simulink library "aeroblk_lib_HL20"  (R2023a)
settings: Solver=ode45  StartTime=0.0  StopTime=10.0  RelTol=1e-3
values from neighbouring files (symbols this model uses):
  alpha_vec_Cn0 = [-10 -5 0 5 10 15 20 25 30]    [aeroblk_init_HL20.m]
  b_ref = 13.89/m2ft    (= 4.23367186452)    [aeroblk_init_HL20.m]
  beta_vec_Cn0 = [0 2 5 10]    [aeroblk_init_HL20.m]
  Clbeta = -0.00787    [aeroblk_init_HL20.m]
  Clda = temp(:,6)    [aeroblk_init_HL20.m]
  Clddf = temp(:,4)    [aeroblk_init_HL20.m]
  Cldr = temp(:,6)    [aeroblk_init_HL20.m]
  Clp = [-4.98 -6.0 -3.98 -5.79 -4.25 -4.99 -6.49 -6.19 -8.10 -8.72 -24.10]*1e-1    [aeroblk_init_HL20.m]
  Clr = [4.96 5.98 8.40 8.06 6.86 5.72 6.03 8.99 9.57 13.57 44.90]*1e-1    [aeroblk_init_HL20.m]
  Cm0 = reshape(temp(:,2),length(beta_vec_0),length(alpha_vec_0))    [aeroblk_init_HL20.m]
  Cmda = temp(:,2)    [aeroblk_init_HL20.m]
  Cmde = temp(:,2)    [aeroblk_init_HL20.m]
  Cmdfn = temp(:,2)    [aeroblk_init_HL20.m]
  Cmdfp = temp(:,2)    [aeroblk_init_HL20.m]
  Cmdr = temp(:,2)    [aeroblk_init_HL20.m]
  Cmq = [-2.03 -1.58 -1.16 -1.76 -1.76 -1.75 -1.74 -2.52 -2.99 -5.71 -8]*1e-1    [aeroblk_init_HL20.m]
  Cn0 = [0 0.46 1.15 2.30 ... (first row only)    [aeroblk_init_HL20.m]
  Cnda = temp(:,5)    [aeroblk_init_HL20.m]
  Cnddf = temp(:,3)    [aeroblk_init_HL20.m]
  Cndr = temp(:,5)    [aeroblk_init_HL20.m]
  Cnp = [3.81 3.53 2.19 2.44 1.79 1.67 2.01 2.22 3.07 3.79 8.50]*1e-1    [aeroblk_init_HL20.m]
  Cnr = [-7.94 -8.37 -9.21 -9.22 -8.67 -9.22 -9.46 -10.07 -10.90 -12.86 -20.41]*1e-1    [aeroblk_init_HL20.m]
  CX0 = -reshape(temp(:,3),length(beta_vec_0),length(alpha_vec_0))    [aeroblk_init_HL20.m]
  CXda = -temp(:,3)    [aeroblk_init_HL20.m]
  CXddf = temp(:,1)    [aeroblk_init_HL20.m]
  CXde = -temp(:,3)    [aeroblk_init_HL20.m]
  CXdfn = -temp(:,3)    [aeroblk_init_HL20.m]
  CXdfp = -temp(:,3)    [aeroblk_init_HL20.m]
  CXdr = -temp(:,3)    [aeroblk_init_HL20.m]
  CYbeta = -0.01242    [aeroblk_init_HL20.m]
  CYda = temp(:,4)    [aeroblk_init_HL20.m]
  CYddf = temp(:,2)    [aeroblk_init_HL20.m]
  CYdr = temp(:,4)    [aeroblk_init_HL20.m]
  CZ0 = -reshape(temp(:,1),length(beta_vec_0),length(alpha_vec_0))    [aeroblk_init_HL20.m]
  CZda = -temp(:,1)    [aeroblk_init_HL20.m]
  CZde = -temp(:,1)    [aeroblk_init_HL20.m]
  CZdfn = -temp(:,1)    [aeroblk_init_HL20.m]
  CZdfp = -temp(:,1)    [aeroblk_init_HL20.m]
  CZdr = -temp(:,1)    [aeroblk_init_HL20.m]
  d_ref = 28.24/m2ft    (= 8.60755172456)    [aeroblk_init_HL20.m]
  mass = massBody+massFuel    (= 11738.9844962)    [aeroblk_init_HL20.m]
  x_cg = 0.575*len_veh    (= 4.78635044684)    [aeroblk_init_HL20.m]
  x_ref = 0.54*len_veh    (= 4.49500737616)    [aeroblk_init_HL20.m]
undefined symbols (not defined in the file or in its folder): a_matrix, A_matrix, b_matrix, B_matrix, c_matrix, C_matrix, d_matrix, F, F_matrix, H_matrix, Kalpha, Kalpha_1, Kbeta, Kbeta_1, Kp, Kp_1, Kphi, Kphi_1, Kq, Kq_1, Kr, Kr_1, Light, MIL
libraries: aerolibschedule x4, aerolibconvert2 x3, aerolibasang x3, aerolibwind2 x3, shared6dof x1, aerolibatmos2 x1, aerolibadyn x1
(part 1 of 2)
Description:
  | HL-20 lifting body and controller library
settings Model: Creator=The MathWorks, Inc.  LastModifiedBy=The MathWorks, Inc.
settings SolverCC: AlgebraicLoopSolver=TrustRegion
settings DataIOCC: LimitDataPoints=on  SaveFormat=Array  SignalLoggingSaveFormat=ModelDataLogs  ReturnWorkspaceOutputs=off
settings OptimizationCC: BlockReduction=off  BooleanDataType=off  ReuseModelBlockBuffer=off  ExpressionDepthLimit=2147483647  LifeSpan=inf
settings DebuggingCC: SaveWithParameterizedLinksMsg=none  UnderspecifiedInitializationDetection=Classic  MergeDetectMultiDrivingBlocksExec=none  SignalResolutionControl=TryResolveAllWithWarning  FcnCallInpInsideContextMsg=warning  UnconnectedInputMsg=warning  UnconnectedOutputMsg=warning  UnconnectedLineMsg=warning  AllowSymbolicDim=off  StateNameClashWarn=warning  SFUnexpectedBacktrackingDiag=warning  SFNoUnconditionalDefaultTransitionDiag=warning  SFExecutionAtInitializationDiag=none  ArithmeticOperatorsInVariantConditions=warning
settings HardwareCC: ProdBitPerPointer=32  ProdBitPerSizeT=32  ProdBitPerPtrDiffT=32  ProdLargestAtomicFloat=None  ProdIntDivRoundTo=Undefined  ProdEndianess=Unspecified  ProdWordSize=32  ProdHWDeviceType=32-bit Generic  TargetUnknown=on
settings ModelReferenceCC: EnableRefExpFcnMdlSchedulingChecks=on  PropagateSignalLabelsOutOfModel=off
settings SFSimCC: SimUseLocalCustomCode=off  CustomCodeUndefinedFunction=UseInterfaceOnly
settings RTWCC: RTWUseLocalCustomCode=off
settings CodeAppCC: StateflowObjectComments=on
settings GRTTargetCC: TargetLangStandard=C89/C90 (ANSI)
settings ConfigComp: CovMetricSettings=dw  CovSaveCumulativeToWorkspaceVar=on  CovSaveSingleToWorkspaceVar=on  CovExternalEMLEnable=off

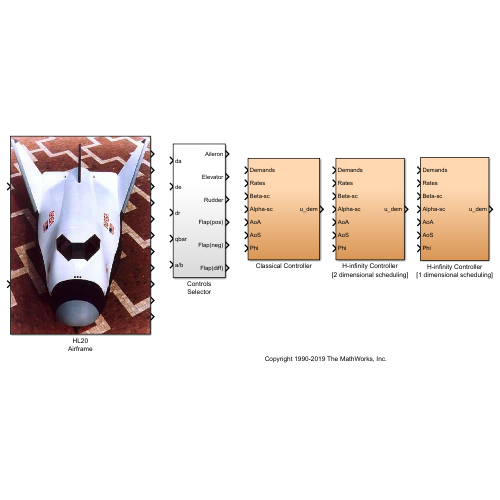
[thumbnail: Simulink's stored preview of the top-level diagram]
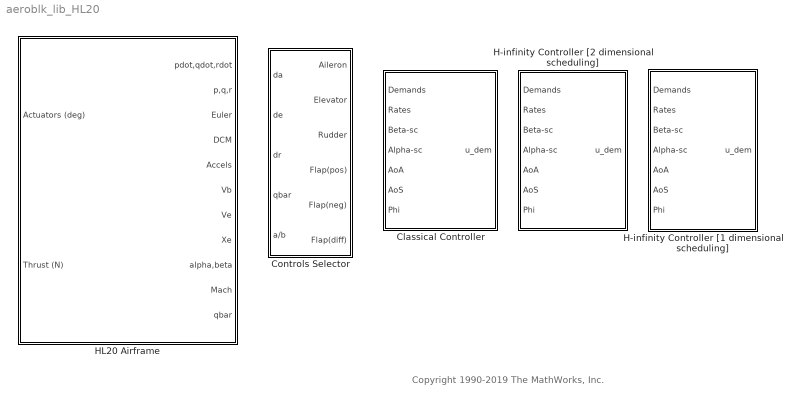
== system aeroblk_lib_HL20 ==
  note: Copyright 1990-2019 The MathWorks, Inc.
  Classical Controller : Subsystem
  Controls Selector : Subsystem
  H-infinity Controller [1 dimensional scheduling] : Subsystem
  H-infinity Controller [2 dimensional scheduling] : Subsystem
  HL20 Airframe : Subsystem
      mask Display: image('aeroblk_HL20pic.jpg')

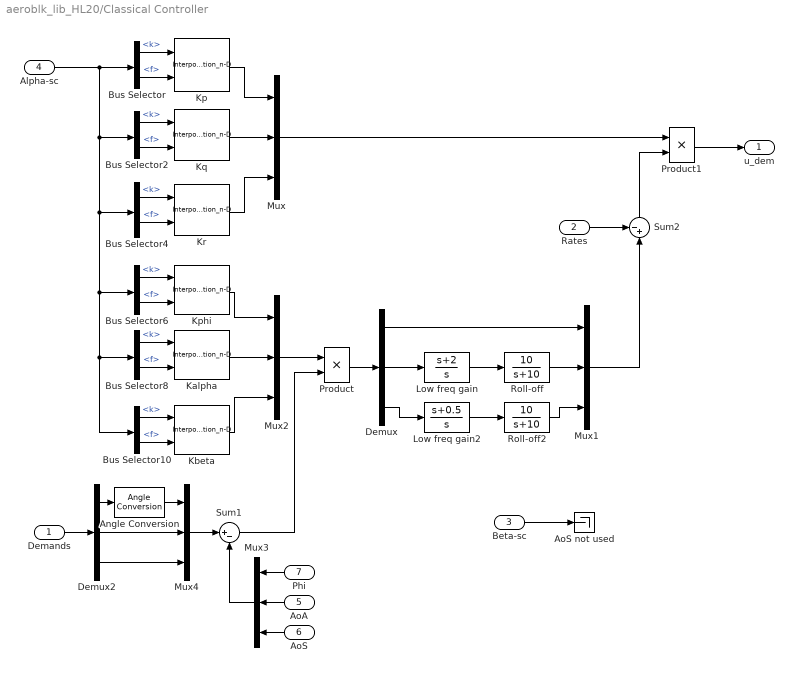
== system aeroblk_lib_HL20/Classical Controller ==
  Demands : Inport  Unit=deg  PortDimensions=3
  Rates : Inport  Port=2  Unit=rad/second  PortDimensions=3
  Beta-sc : Inport  Port=3
  Alpha-sc : Inport  Port=4
  AoA : Inport  Port=5  Unit=deg  PortDimensions=1
  AoS : Inport  Port=6  Unit=deg  PortDimensions=1
  Phi : Inport  Port=7  Unit=rad  PortDimensions=1
  Angle Conversion : aerolibconvert2/Angle Conversion  IU=deg  OU=rad
  AoS not used : Terminator
  Bus Selector{,2,4,6,8,10} (6 alike) : BusSelector  OutputSignals=k,f
  Demux : Demux  Outputs=3
      settings: DisplayOption=none
  Demux2 : Demux  Outputs=3
      settings: DisplayOption=none
  Kalpha : Interpolation_n-D  NumberOfTableDimensions=1  Table=Kalpha_1  RemoveProtectionIndex=on
      settings: InputPortMap=u0,u1
  Kbeta : Interpolation_n-D  NumberOfTableDimensions=1  Table=Kbeta_1  RemoveProtectionIndex=on
      settings: InputPortMap=u0,u1
  Kp : Interpolation_n-D  NumberOfTableDimensions=1  Table=Kp_1  RemoveProtectionIndex=on
      settings: InputPortMap=u0,u1
  Kphi : Interpolation_n-D  NumberOfTableDimensions=1  Table=Kphi_1  RemoveProtectionIndex=on
      settings: InputPortMap=u0,u1
  Kq : Interpolation_n-D  NumberOfTableDimensions=1  Table=Kq_1  RemoveProtectionIndex=on
      settings: InputPortMap=u0,u1
  Kr : Interpolation_n-D  NumberOfTableDimensions=1  Table=Kr_1  RemoveProtectionIndex=on
      settings: InputPortMap=u0,u1
  Low freq gain : TransferFcn  Numerator=[1 2]  Denominator=[1 0]
  Low freq gain2 : TransferFcn  Numerator=[1 0.5]  Denominator=[1 0]
  Mux{,1,3..4} (4 alike) : Mux  Inputs=[1,1,1]
  Mux2 : Mux  Inputs=3
  Product : Product  InputSameDT=on  SaturateOnIntegerOverflow=on  OutDataTypeStr=Inherit: Same as first input
  Product1 : Product  InputSameDT=on  SaturateOnIntegerOverflow=on  OutDataTypeStr=Inherit: Same as first input
  Roll-off : TransferFcn  Numerator=10  Denominator=[1 10]
  Roll-off2 : TransferFcn  Numerator=10  Denominator=[1 10]
  Sum1 : Sum  Inputs=|+-  InputSameDT=on  SaturateOnIntegerOverflow=on  OutDataTypeStr=Inherit: Same as first input
  Sum2 : Sum  Inputs=-+|  InputSameDT=on  SaturateOnIntegerOverflow=on  OutDataTypeStr=Inherit: Same as first input
  u_dem : Outport  OutputWhenDisabled=reset  InitialOutput=[0 0 0]  VectorParamsAs1DForOutWhenUnconnected=off
  wires:
  Beta-sc/1 -> AoS not used/1
  Product1/1 -> u_dem/1
  Mux4/1 -> Sum1/1
  Demux2/3 -> Mux4/3
  Demux2/2 -> Mux4/2
  Angle Conversion/1 -> Mux4/1
  Demux2/1 -> Angle Conversion/1
  Demands/1 -> Demux2/1
  Kphi/1 -> Mux2/1
  Kbeta/1 -> Mux2/3
  Kalpha/1 -> Mux2/2
  Mux1/1 -> Sum2/2
  Sum2/1 -> Product1/2
  Mux/1 -> Product1/1
  Rates/1 -> Sum2/1
  Demux/1 -> Mux1/1
  Roll-off2/1 -> Mux1/3
  Roll-off/1 -> Mux1/2
  Demux/3 -> Low freq gain2/1
  Demux/2 -> Low freq gain/1
  Product/1 -> Demux/1
  Sum1/1 -> Product/2
  Mux2/1 -> Product/1
  AoS/1 -> Mux3/3
  AoA/1 -> Mux3/2
  Phi/1 -> Mux3/1
  Mux3/1 -> Sum1/2
  Low freq gain/1 -> Roll-off/1
  Low freq gain2/1 -> Roll-off2/1
  Kr/1 -> Mux/3
  Kp/1 -> Mux/1
  Kq/1 -> Mux/2
  Bus Selector/1 -> Kp/1  "<k>"
  Bus Selector/2 -> Kp/2  "<f>"
  Bus Selector2/1 -> Kq/1  "<k>"
  Bus Selector2/2 -> Kq/2  "<f>"
  Bus Selector4/1 -> Kr/1  "<k>"
  Bus Selector4/2 -> Kr/2  "<f>"
  Bus Selector6/1 -> Kphi/1  "<k>"
  Bus Selector6/2 -> Kphi/2  "<f>"
  Bus Selector8/1 -> Kalpha/1  "<k>"
  Bus Selector10/1 -> Kbeta/1  "<k>"
  Bus Selector10/2 -> Kbeta/2  "<f>"
  Bus Selector8/2 -> Kalpha/2  "<f>"
  Alpha-sc/1 -> Bus Selector/1, Bus Selector2/1, Bus Selector4/1, Bus Selector6/1, Bus Selector8/1, Bus Selector10/1

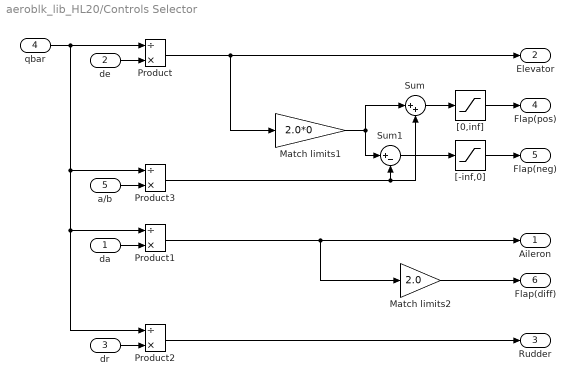
== system aeroblk_lib_HL20/Controls Selector ==
  da : Inport
  de : Inport  Port=2
  dr : Inport  Port=3
  qbar : Inport  Port=4  Unit=pascal
  a/b : Inport  Port=5
  Match limits1 : Gain  Gain=2.0*0  SaturateOnIntegerOverflow=on  OutDataTypeStr=Inherit: Same as input  ParamDataTypeStr=Inherit: Same as input
  Match limits2 : Gain  Gain=2.0  SaturateOnIntegerOverflow=on  OutDataTypeStr=Inherit: Same as input  ParamDataTypeStr=Inherit: Same as input
  Product{,1..3} (4 alike) : Product  Inputs=/*  InputSameDT=on  SaturateOnIntegerOverflow=on  OutDataTypeStr=Inherit: Same as first input
  Sum : Sum  Inputs=|++  InputSameDT=on  SaturateOnIntegerOverflow=on  OutDataTypeStr=Inherit: Same as first input
  Sum1 : Sum  Inputs=|+-  InputSameDT=on  SaturateOnIntegerOverflow=on  OutDataTypeStr=Inherit: Same as first input
  "[-inf,0]" : Saturate  UpperLimit=0  LowerLimit=-inf
  "[0,inf]" : Saturate  UpperLimit=inf  LowerLimit=0
  Aileron : Outport  Unit=deg  VectorParamsAs1DForOutWhenUnconnected=off
  Elevator : Outport  Port=2  Unit=deg  VectorParamsAs1DForOutWhenUnconnected=off
  Rudder : Outport  Port=3  Unit=deg  VectorParamsAs1DForOutWhenUnconnected=off
  Flap(pos) : Outport  Port=4  Unit=deg  VectorParamsAs1DForOutWhenUnconnected=off
  Flap(neg) : Outport  Port=5  Unit=deg  VectorParamsAs1DForOutWhenUnconnected=off
  Flap(diff) : Outport  Port=6  Unit=deg  VectorParamsAs1DForOutWhenUnconnected=off
  wires:
  qbar/1 -> Product/1, Product2/1, Product1/1, Product3/1
  de/1 -> Product/2
  Product2/1 -> Rudder/1
  dr/1 -> Product2/2
  da/1 -> Product1/2
  Product1/1 -> Match limits2/1, Aileron/1
  Product/1 -> Elevator/1, Match limits1/1
  Match limits1/1 -> Sum/1, Sum1/1
  "[-inf,0]"/1 -> Flap(neg)/1
  "[0,inf]"/1 -> Flap(pos)/1
  Match limits2/1 -> Flap(diff)/1
  a/b/1 -> Product3/2
  Sum/1 -> "[0,inf]"/1
  Sum1/1 -> "[-inf,0]"/1
  Product3/1 -> Sum1/2, Sum/2

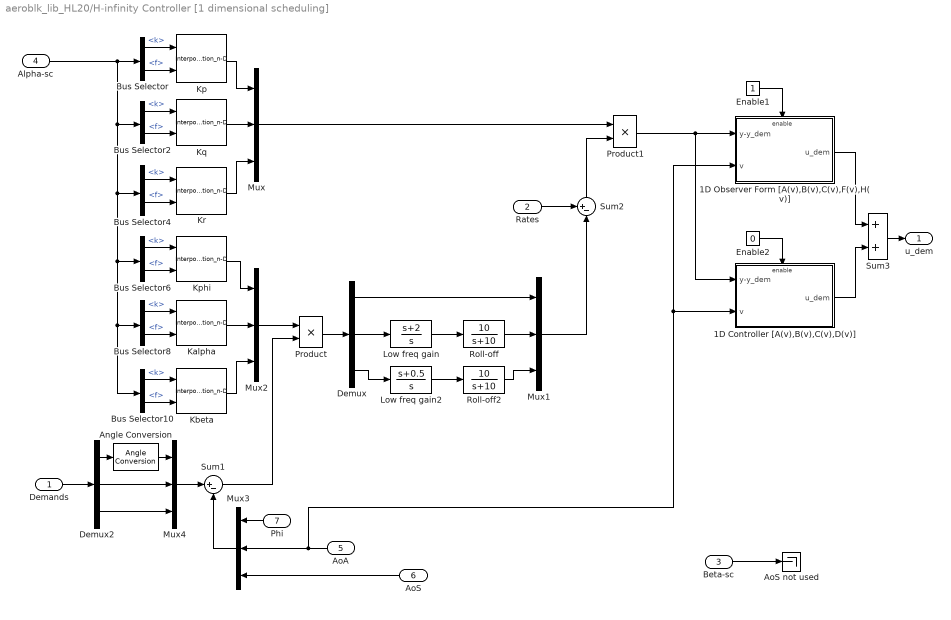
== system aeroblk_lib_HL20/H-infinity Controller [1 dimensional scheduling] ==
  Demands : Inport  Unit=deg  PortDimensions=3
  Rates : Inport  Port=2  Unit=rad/second  PortDimensions=3
  Beta-sc : Inport  Port=3
  Alpha-sc : Inport  Port=4
  AoA : Inport  Port=5  Unit=deg  PortDimensions=1
  AoS : Inport  Port=6  Unit=deg  PortDimensions=1
  Phi : Inport  Port=7  Unit=radian  PortDimensions=1
  1D Controller [A(v),B(v),C(v),D(v)] : Subsystem  TreatAsAtomicUnit=on
  1D Observer Form [A(v),B(v),C(v),F(v),H(v)] : Subsystem  TreatAsAtomicUnit=on
  Angle Conversion : aerolibconvert2/Angle Conversion  IU=deg  OU=rad
  AoS not used : Terminator
  Bus Selector{,2,4,6,8,10} (6 alike) : BusSelector  OutputSignals=k,f
  Demux : Demux  Outputs=3
      settings: DisplayOption=none
  Demux2 : Demux  Outputs=3
      settings: DisplayOption=none
  Enable1 : Constant
  Enable2 : Constant  Value=0
  Kalpha : Interpolation_n-D  NumberOfTableDimensions=1  Table=Kalpha_1  RemoveProtectionIndex=on
      settings: InputPortMap=u0,u1
  Kbeta : Interpolation_n-D  NumberOfTableDimensions=1  Table=Kbeta_1  RemoveProtectionIndex=on
      settings: InputPortMap=u0,u1
  Kp : Interpolation_n-D  NumberOfTableDimensions=1  Table=Kp_1  RemoveProtectionIndex=on
      settings: InputPortMap=u0,u1
  Kphi : Interpolation_n-D  NumberOfTableDimensions=1  Table=Kphi_1  RemoveProtectionIndex=on
      settings: InputPortMap=u0,u1
  Kq : Interpolation_n-D  NumberOfTableDimensions=1  Table=Kq_1  RemoveProtectionIndex=on
      settings: InputPortMap=u0,u1
  Kr : Interpolation_n-D  NumberOfTableDimensions=1  Table=Kr_1  RemoveProtectionIndex=on
      settings: InputPortMap=u0,u1
  Low freq gain : TransferFcn  Numerator=[1 2]  Denominator=[1 0]
  Low freq gain2 : TransferFcn  Numerator=[1 0.5]  Denominator=[1 0]
  Mux{,1,3..4} (4 alike) : Mux  Inputs=[1,1,1]
  Mux2 : Mux  Inputs=3
  Product : Product  InputSameDT=on  SaturateOnIntegerOverflow=on  OutDataTypeStr=Inherit: Same as first input
  Product1 : Product  InputSameDT=on  SaturateOnIntegerOverflow=on  OutDataTypeStr=Inherit: Same as first input
  Roll-off : TransferFcn  Numerator=10  Denominator=[1 10]
  Roll-off2 : TransferFcn  Numerator=10  Denominator=[1 10]
  Sum1 : Sum  Inputs=|+-  InputSameDT=on  SaturateOnIntegerOverflow=on  OutDataTypeStr=Inherit: Same as first input
  Sum2 : Sum  Inputs=+-|  InputSameDT=on  SaturateOnIntegerOverflow=on  OutDataTypeStr=Inherit: Same as first input
  Sum3 : Sum  InputSameDT=on  SaturateOnIntegerOverflow=on  OutDataTypeStr=Inherit: Same as first input
  u_dem : Outport  OutputWhenDisabled=reset  InitialOutput=[0 0 0]  VectorParamsAs1DForOutWhenUnconnected=off
  wires:
  Beta-sc/1 -> AoS not used/1
  Mux4/1 -> Sum1/1
  Demux2/3 -> Mux4/3
  Demux2/2 -> Mux4/2
  Angle Conversion/1 -> Mux4/1
  Demux2/1 -> Angle Conversion/1
  Demands/1 -> Demux2/1
  Mux1/1 -> Sum2/2
  Sum2/1 -> Product1/2
  Mux/1 -> Product1/1
  Rates/1 -> Sum2/1
  Demux/1 -> Mux1/1
  Roll-off2/1 -> Mux1/3
  Roll-off/1 -> Mux1/2
  Demux/3 -> Low freq gain2/1
  Demux/2 -> Low freq gain/1
  Product/1 -> Demux/1
  Sum1/1 -> Product/2
  Mux2/1 -> Product/1
  AoS/1 -> Mux3/3
  AoA/1 -> 1D Observer Form [A(v),B(v),C(v),F(v),H(v)]/2(v), 1D Controller [A(v),B(v),C(v),D(v)]/2(v), Mux3/2
  Phi/1 -> Mux3/1
  Mux3/1 -> Sum1/2
  Low freq gain/1 -> Roll-off/1
  Low freq gain2/1 -> Roll-off2/1
  Alpha-sc/1 -> Bus Selector8/1, Bus Selector10/1, Bus Selector6/1, Bus Selector4/1, Bus Selector2/1, Bus Selector/1
  Product1/1 -> 1D Observer Form [A(v),B(v),C(v),F(v),H(v)]/1(y-y_dem), 1D Controller [A(v),B(v),C(v),D(v)]/1(y-y_dem)
  Enable1/1 -> 1D Observer Form [A(v),B(v),C(v),F(v),H(v)]/Enable
  Enable2/1 -> 1D Controller [A(v),B(v),C(v),D(v)]/Enable
  1D Observer Form [A(v),B(v),C(v),F(v),H(v)]/1(u_dem) -> Sum3/1
  1D Controller [A(v),B(v),C(v),D(v)]/1(u_dem) -> Sum3/2
  Sum3/1 -> u_dem/1
  Bus Selector8/2 -> Kalpha/2  "<f>"
  Bus Selector10/2 -> Kbeta/2  "<f>"
  Bus Selector10/1 -> Kbeta/1  "<k>"
  Bus Selector8/1 -> Kalpha/1  "<k>"
  Bus Selector6/2 -> Kphi/2  "<f>"
  Bus Selector6/1 -> Kphi/1  "<k>"
  Bus Selector4/2 -> Kr/2  "<f>"
  Bus Selector4/1 -> Kr/1  "<k>"
  Bus Selector2/2 -> Kq/2  "<f>"
  Bus Selector2/1 -> Kq/1  "<k>"
  Bus Selector/2 -> Kp/2  "<f>"
  Bus Selector/1 -> Kp/1  "<k>"
  Kp/1 -> Mux/1
  Kq/1 -> Mux/2
  Kr/1 -> Mux/3
  Kphi/1 -> Mux2/1
  Kbeta/1 -> Mux2/3
  Kalpha/1 -> Mux2/2

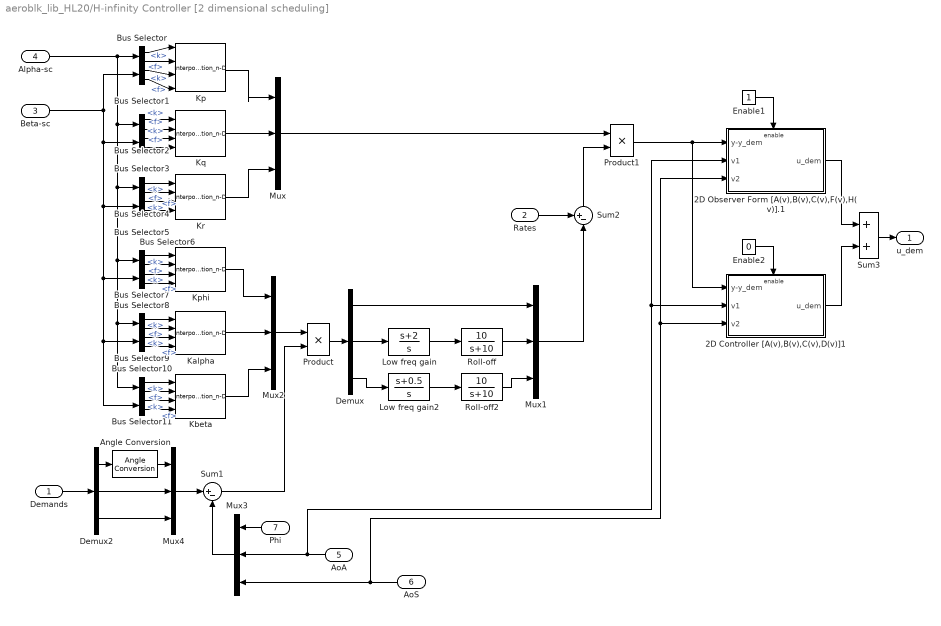
== system aeroblk_lib_HL20/H-infinity Controller [2 dimensional scheduling] ==
  Demands : Inport  Unit=degree  PortDimensions=3
  Rates : Inport  Port=2  Unit=rad/second  PortDimensions=3
  Beta-sc : Inport  Port=3
  Alpha-sc : Inport  Port=4
  AoA : Inport  Port=5  Unit=deg  PortDimensions=1
  AoS : Inport  Port=6  Unit=deg  PortDimensions=1
  Phi : Inport  Port=7  Unit=radian  PortDimensions=1
  2D Controller [A(v),B(v),C(v),D(v)]1 : Subsystem  TreatAsAtomicUnit=on
  2D Observer Form [A(v),B(v),C(v),F(v),H(v)].1 : Subsystem  TreatAsAtomicUnit=on
  Angle Conversion : aerolibconvert2/Angle Conversion  IU=deg  OU=rad
  Bus Selector{,1..11} (12 alike) : BusSelector  OutputSignals=k,f
  Demux : Demux  Outputs=3
      settings: DisplayOption=none
  Demux2 : Demux  Outputs=3
      settings: DisplayOption=none
  Enable1 : Constant
  Enable2 : Constant  Value=0
  Kalpha : Interpolation_n-D  Table=Kalpha  RemoveProtectionIndex=on
  Kbeta : Interpolation_n-D  Table=Kbeta  RemoveProtectionIndex=on
  Kp : Interpolation_n-D  Table=Kp  RemoveProtectionIndex=on
  Kphi : Interpolation_n-D  Table=Kphi  RemoveProtectionIndex=on
  Kq : Interpolation_n-D  Table=Kq  RemoveProtectionIndex=on
  Kr : Interpolation_n-D  Table=Kr  RemoveProtectionIndex=on
  Low freq gain : TransferFcn  Numerator=[1 2]  Denominator=[1 0]
  Low freq gain2 : TransferFcn  Numerator=[1 0.5]  Denominator=[1 0]
  Mux{,1,3..4} (4 alike) : Mux  Inputs=[1,1,1]
  Mux2 : Mux  Inputs=3
  Product : Product  InputSameDT=on  SaturateOnIntegerOverflow=on  OutDataTypeStr=Inherit: Same as first input
  Product1 : Product  InputSameDT=on  SaturateOnIntegerOverflow=on  OutDataTypeStr=Inherit: Same as first input
  Roll-off : TransferFcn  Numerator=10  Denominator=[1 10]
  Roll-off2 : TransferFcn  Numerator=10  Denominator=[1 10]
  Sum1 : Sum  Inputs=|+-  InputSameDT=on  SaturateOnIntegerOverflow=on  OutDataTypeStr=Inherit: Same as first input
  Sum2 : Sum  Inputs=+-|  InputSameDT=on  SaturateOnIntegerOverflow=on  OutDataTypeStr=Inherit: Same as first input
  Sum3 : Sum  InputSameDT=on  SaturateOnIntegerOverflow=on  OutDataTypeStr=Inherit: Same as first input
  u_dem : Outport  OutputWhenDisabled=reset  InitialOutput=[0 0 0]  VectorParamsAs1DForOutWhenUnconnected=off
  wires:
  Sum3/1 -> u_dem/1
  2D Controller [A(v),B(v),C(v),D(v)]1/1(u_dem) -> Sum3/2
  2D Observer Form [A(v),B(v),C(v),F(v),H(v)].1/1(u_dem) -> Sum3/1
  Enable2/1 -> 2D Controller [A(v),B(v),C(v),D(v)]1/Enable
  Enable1/1 -> 2D Observer Form [A(v),B(v),C(v),F(v),H(v)].1/Enable
  Product1/1 -> 2D Observer Form [A(v),B(v),C(v),F(v),H(v)].1/1(y-y_dem), 2D Controller [A(v),B(v),C(v),D(v)]1/1(y-y_dem)
  Beta-sc/1 -> Bus Selector9/1, Bus Selector11/1, Bus Selector7/1, Bus Selector5/1, Bus Selector3/1, Bus Selector1/1
  Alpha-sc/1 -> Bus Selector8/1, Bus Selector10/1, Bus Selector6/1, Bus Selector4/1, Bus Selector2/1, Bus Selector/1
  Kq/1 -> Mux/2
  Kp/1 -> Mux/1
  Kr/1 -> Mux/3
  Low freq gain2/1 -> Roll-off2/1
  Low freq gain/1 -> Roll-off/1
  Mux3/1 -> Sum1/2
  Phi/1 -> Mux3/1
  AoA/1 -> 2D Observer Form [A(v),B(v),C(v),F(v),H(v)].1/2(v1), 2D Controller [A(v),B(v),C(v),D(v)]1/2(v1), Mux3/2
  AoS/1 -> 2D Observer Form [A(v),B(v),C(v),F(v),H(v)].1/3(v2), 2D Controller [A(v),B(v),C(v),D(v)]1/3(v2), Mux3/3
  Mux2/1 -> Product/1
  Sum1/1 -> Product/2
  Product/1 -> Demux/1
  Demux/2 -> Low freq gain/1
  Demux/3 -> Low freq gain2/1
  Roll-off/1 -> Mux1/2
  Roll-off2/1 -> Mux1/3
  Demux/1 -> Mux1/1
  Rates/1 -> Sum2/1
  Mux/1 -> Product1/1
  Sum2/1 -> Product1/2
  Mux1/1 -> Sum2/2
  Kalpha/1 -> Mux2/2
  Kbeta/1 -> Mux2/3
  Kphi/1 -> Mux2/1
  Demands/1 -> Demux2/1
  Demux2/1 -> Angle Conversion/1
  Angle Conversion/1 -> Mux4/1
  Demux2/2 -> Mux4/2
  Demux2/3 -> Mux4/3
  Mux4/1 -> Sum1/1
  Bus Selector/1 -> Kp/1  "<k>"
  Bus Selector/2 -> Kp/2  "<f>"
  Bus Selector1/1 -> Kp/3  "<k>"
  Bus Selector1/2 -> Kp/4  "<f>"
  Bus Selector2/1 -> Kq/1  "<k>"
  Bus Selector2/2 -> Kq/2  "<f>"
  Bus Selector3/1 -> Kq/3  "<k>"
  Bus Selector3/2 -> Kq/4  "<f>"
  Bus Selector4/1 -> Kr/1  "<k>"
  Bus Selector4/2 -> Kr/2  "<f>"
  Bus Selector5/1 -> Kr/3  "<k>"
  Bus Selector5/2 -> Kr/4  "<f>"
  Bus Selector6/1 -> Kphi/1  "<k>"
  Bus Selector6/2 -> Kphi/2  "<f>"
  Bus Selector7/1 -> Kphi/3  "<k>"
  Bus Selector7/2 -> Kphi/4  "<f>"
  Bus Selector8/1 -> Kalpha/1  "<k>"
  Bus Selector8/2 -> Kalpha/2  "<f>"
  Bus Selector9/1 -> Kalpha/3  "<k>"
  Bus Selector9/2 -> Kalpha/4  "<f>"
  Bus Selector10/1 -> Kbeta/1  "<k>"
  Bus Selector10/2 -> Kbeta/2  "<f>"
  Bus Selector11/1 -> Kbeta/3  "<k>"
  Bus Selector11/2 -> Kbeta/4  "<f>"

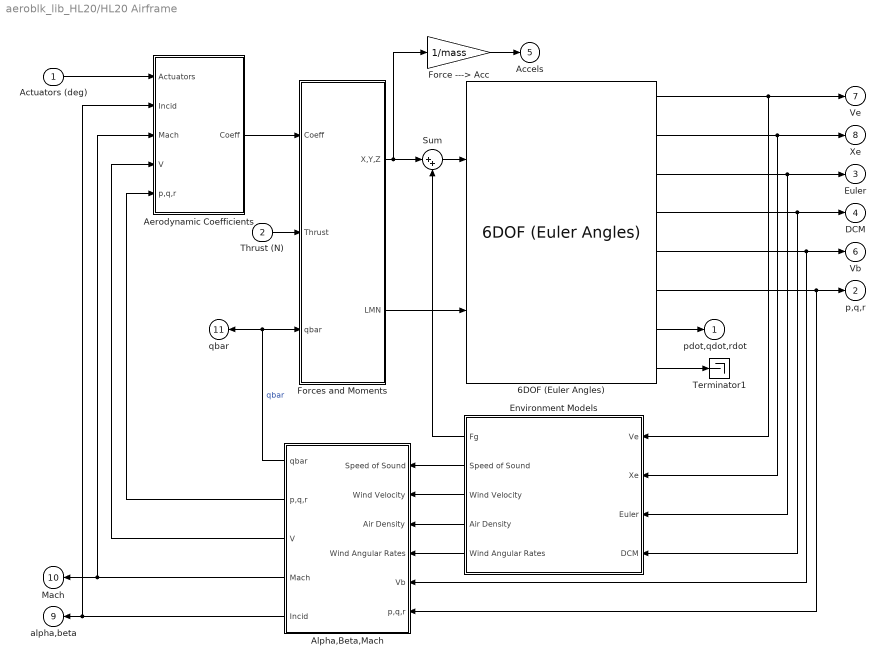
== system aeroblk_lib_HL20/HL20 Airframe ==
  Actuators (deg) : Inport  Unit=deg
  Thrust (N) : Inport  Port=2  Unit=N
  6DOF (Euler Angles) : shared6dof/6DOF (Euler Angles)  units=Metric (MKS)  mtype=Fixed  rep=Euler Angles  xme_0=xme_0  Vm_0=Vmw  eul_0=Euler_0  pm_0=pm_0  mass_0=mass  mass_e=0.5  mass_f=2.0  inertia=Inertia  inertia_e=eye(3)  inertia_f=2*eye(3)  k_quat=1.0  vre_flag=on  abi_flag=off  aMode=aMode  xme_statename=''  Vm_statename=''  eul_statename=''  quat_statename=''  pm_statename=''  mass_statename=''
  Aerodynamic Coefficients : Subsystem
  Alpha,Beta,Mach : Subsystem
  Environment Models : Subsystem
  Force ---> Acc : Gain  Gain=1/mass  SaturateOnIntegerOverflow=on  OutDataTypeStr=Inherit: Same as input  ParamDataTypeStr=Inherit: Same as input
  Forces and Moments : Subsystem
  Sum : Sum  Inputs=|++  InputSameDT=on  SaturateOnIntegerOverflow=on  OutDataTypeStr=Inherit: Same as first input
  Terminator1 : Terminator
  pdot,qdot,rdot : Outport  Unit=rad/s^2  InitialOutput=0  VectorParamsAs1DForOutWhenUnconnected=off
  p,q,r : Outport  Port=2  Unit=rad/second  InitialOutput=0  VectorParamsAs1DForOutWhenUnconnected=off
  Euler : Outport  Port=3  Unit=rad  InitialOutput=0  VectorParamsAs1DForOutWhenUnconnected=off
  DCM : Outport  Port=4  InitialOutput=0  VectorParamsAs1DForOutWhenUnconnected=off
  Accels : Outport  Port=5  Unit=m/s^2  InitialOutput=0  VectorParamsAs1DForOutWhenUnconnected=off
  Vb : Outport  Port=6  Unit=m/second  InitialOutput=0  VectorParamsAs1DForOutWhenUnconnected=off
  Ve : Outport  Port=7  Unit=m/s  InitialOutput=0  VectorParamsAs1DForOutWhenUnconnected=off
  Xe : Outport  Port=8  Unit=meter  InitialOutput=0  VectorParamsAs1DForOutWhenUnconnected=off
  alpha,beta : Outport  Port=9  Unit=rad  InitialOutput=0  VectorParamsAs1DForOutWhenUnconnected=off
  Mach : Outport  Port=10  InitialOutput=0  VectorParamsAs1DForOutWhenUnconnected=off
  qbar : Outport  Port=11  Unit=Pa  InitialOutput=0  VectorParamsAs1DForOutWhenUnconnected=off
  wires:
  Environment Models/5(Wind Angular Rates) -> Alpha,Beta,Mach/4(Wind Angular Rates)
  Alpha,Beta,Mach/2("p,q,r ") -> Aerodynamic Coefficients/5(p,q,r)
  Alpha,Beta,Mach/4(Mach) -> Mach/1, Aerodynamic Coefficients/3(Mach)
  Alpha,Beta,Mach/3(V) -> Aerodynamic Coefficients/4(V)
  Actuators (deg)/1 -> Aerodynamic Coefficients/1(Actuators)
  Force ---> Acc/1 -> Accels/1
  Environment Models/1(Fg) -> Sum/2
  Sum/1 -> 6DOF (Euler Angles)/1
  Forces and Moments/1(X,Y,Z) -> Sum/1, Force ---> Acc/1
  Alpha,Beta,Mach/1(qbar) -> qbar/1, Forces and Moments/3(qbar)  "qbar"
  Forces and Moments/2(LMN) -> 6DOF (Euler Angles)/2
  Environment Models/4(Air Density) -> Alpha,Beta,Mach/3(Air Density)
  Environment Models/2(Speed of Sound) -> Alpha,Beta,Mach/1(Speed of Sound)
  6DOF (Euler Angles)/5 -> Vb/1, Alpha,Beta,Mach/5(Vb)
  Environment Models/3(Wind Velocity) -> Alpha,Beta,Mach/2(Wind Velocity)
  Aerodynamic Coefficients/1(Coeff) -> Forces and Moments/1(Coeff)
  Alpha,Beta,Mach/5(Incid) -> Aerodynamic Coefficients/2(Incid), alpha,beta/1
  6DOF (Euler Angles)/3 -> Euler/1, Environment Models/3(Euler)
  6DOF (Euler Angles)/4 -> Environment Models/4(DCM), DCM/1
  6DOF (Euler Angles)/7 -> pdot,qdot,rdot/1
  Thrust (N)/1 -> Forces and Moments/2(Thrust)
  6DOF (Euler Angles)/6 -> Alpha,Beta,Mach/6(p,q,r), p,q,r/1
  6DOF (Euler Angles)/2 -> Xe/1, Environment Models/2(Xe)
  6DOF (Euler Angles)/1 -> Ve/1, Environment Models/1(Ve)
  6DOF (Euler Angles)/8 -> Terminator1/1

== system aeroblk_lib_HL20/H-infinity Controller [1 dimensional scheduling]/1D Controller [A(v),B(v),C(v),D(v)] ==
  y-y_dem : Inport  PortDimensions=3
  v : Inport  Port=2  PortDimensions=1
  Enable : EnablePort
  -1 : Gain  Gain=-1  SaturateOnIntegerOverflow=on  OutDataTypeStr=Inherit: Same as input  ParamDataTypeStr=Inherit: Same as input
  1D Controller [A(v),B(v),C(v),D(v)] : aerolibschedule/1D Controller [A(v),B(v),C(v),D(v)]  A=squeeze(a_matrix(:,:,:,3))  B=squeeze(b_matrix(:,:,:,3))  C=squeeze(c_matrix(:,:,:,3))  D=squeeze(d_matrix(:,:,:,3))  AoA_vec=a_vec  x_initial=0
  u_dem : Outport  OutputWhenDisabled=reset  InitialOutput=[0 0 0]  VectorParamsAs1DForOutWhenUnconnected=off
  wires:
  y-y_dem/1 -> -1/1
  -1/1 -> 1D Controller [A(v),B(v),C(v),D(v)]/1
  1D Controller [A(v),B(v),C(v),D(v)]/1 -> u_dem/1
  v/1 -> 1D Controller [A(v),B(v),C(v),D(v)]/2

== system aeroblk_lib_HL20/H-infinity Controller [1 dimensional scheduling]/1D Observer Form [A(v),B(v),C(v),F(v),H(v)] ==
  y-y_dem : Inport  PortDimensions=3
  v : Inport  Port=2  PortDimensions=1
  Enable : EnablePort
  1D Observer Form [A(v),B(v),C(v),F(v),H(v)] : aerolibschedule/1D Observer Form [A(v),B(v),C(v),F(v),H(v)]  A=squeeze(A_matrix(:,:,:,3))  B=squeeze(B_matrix(:,:,:,3))  C=squeeze(C_matrix(:,:,:,3))  F=squeeze(F_matrix(:,:,:,3))  H=squeeze(H_matrix(:,:,:,3))  AoA_vec=a_vec  x_initial=0
  Signal Specification : SignalSpecification  Dimensions=3
  u_dem : Outport  OutputWhenDisabled=reset  InitialOutput=[0 0 0]  VectorParamsAs1DForOutWhenUnconnected=off
  wires:
  y-y_dem/1 -> 1D Observer Form [A(v),B(v),C(v),F(v),H(v)]/1
  v/1 -> 1D Observer Form [A(v),B(v),C(v),F(v),H(v)]/2
  1D Observer Form [A(v),B(v),C(v),F(v),H(v)]/1 -> Signal Specification/1
  Signal Specification/1 -> 1D Observer Form [A(v),B(v),C(v),F(v),H(v)]/3, u_dem/1

== system aeroblk_lib_HL20/H-infinity Controller [2 dimensional scheduling]/2D Controller [A(v),B(v),C(v),D(v)]1 ==
  y-y_dem : Inport  PortDimensions=3
  v1 : Inport  Port=2  PortDimensions=1
  v2 : Inport  Port=3  PortDimensions=1
  Enable : EnablePort
  -1 : Gain  Gain=-1  SaturateOnIntegerOverflow=on  OutDataTypeStr=Inherit: Same as input  ParamDataTypeStr=Inherit: Same as input
  2D Controller [A(v),B(v),C(v),D(v)]1 : aerolibschedule/2D Controller [A(v),B(v),C(v),D(v)]  A=a_matrix  B=b_matrix  C=c_matrix  D=d_matrix  AoA_vec=a_vec  Mach_vec=b_vec  x_initial=0
  u_dem : Outport  OutputWhenDisabled=reset  InitialOutput=[0 0 0]  VectorParamsAs1DForOutWhenUnconnected=off
  wires:
  v2/1 -> 2D Controller [A(v),B(v),C(v),D(v)]1/3
  v1/1 -> 2D Controller [A(v),B(v),C(v),D(v)]1/2
  2D Controller [A(v),B(v),C(v),D(v)]1/1 -> u_dem/1
  -1/1 -> 2D Controller [A(v),B(v),C(v),D(v)]1/1
  y-y_dem/1 -> -1/1

== system aeroblk_lib_HL20/H-infinity Controller [2 dimensional scheduling]/2D Observer Form [A(v),B(v),C(v),F(v),H(v)].1 ==
  y-y_dem : Inport  PortDimensions=3
  v1 : Inport  Port=2  PortDimensions=1
  v2 : Inport  Port=3  PortDimensions=1
  Enable : EnablePort
  2D Observer Form [A(v),B(v),C(v),F(v),H(v)] : aerolibschedule/2D Observer Form [A(v),B(v),C(v),F(v),H(v)]  A=A_matrix  B=B_matrix  C=C_matrix  F=F_matrix  H=H_matrix  AoA_vec=a_vec  Mach_vec=b_vec  x_initial=0
  Signal Specification : SignalSpecification  Dimensions=3
  u_dem : Outport  OutputWhenDisabled=reset  InitialOutput=[0 0 0]  VectorParamsAs1DForOutWhenUnconnected=off
  wires:
  Signal Specification/1 -> 2D Observer Form [A(v),B(v),C(v),F(v),H(v)]/4, u_dem/1
  2D Observer Form [A(v),B(v),C(v),F(v),H(v)]/1 -> Signal Specification/1
  v2/1 -> 2D Observer Form [A(v),B(v),C(v),F(v),H(v)]/3
  v1/1 -> 2D Observer Form [A(v),B(v),C(v),F(v),H(v)]/2
  y-y_dem/1 -> 2D Observer Form [A(v),B(v),C(v),F(v),H(v)]/1

== system aeroblk_lib_HL20/HL20 Airframe/Aerodynamic Coefficients ==
  Actuators : Inport  Unit=deg
  Incid : Inport  Port=2  Unit=rad
  Mach : Inport  Port=3
  V : Inport  Port=4  Unit=m/s
  p,q,r : Inport  Port=5  Unit=rad/second
  Actuator Increments : Subsystem
  Body Rate Damping : Subsystem
  Datum Coefficients : Subsystem
  Demux : Demux  Outputs=2
      settings: DisplayOption=none
  Sum1 : Sum  Inputs=+++  InputSameDT=on  SaturateOnIntegerOverflow=on  OutDataTypeStr=Inherit: Same as first input
  Terminator2 : Terminator
  Unit Conversion : UnitConversion
  Coeff : Outport  InitialOutput=0  VectorParamsAs1DForOutWhenUnconnected=off
  wires:
  Demux/1 -> Datum Coefficients/1(Alpha), Actuator Increments/1(Alpha), Body Rate Damping/3(Alpha)
  p,q,r/1 -> Body Rate Damping/2(p,q,r)
  Incid/1 -> Unit Conversion/1
  Unit Conversion/1 -> Demux/1
  Actuators/1 -> Actuator Increments/3("Actuator Deflections ")
  Sum1/1 -> Coeff/1
  Datum Coefficients/1(cl) -> Sum1/2
  Demux/2 -> Datum Coefficients/2(Beta), Actuator Increments/2(Beta)
  Mach/1 -> Terminator2/1
  V/1 -> Body Rate Damping/1(V)
  Body Rate Damping/1(cl) -> Sum1/1
  Actuator Increments/1(cl) -> Sum1/3

== system aeroblk_lib_HL20/HL20 Airframe/Alpha,Beta,Mach ==
  Speed of Sound : Inport  Unit=m/s
  Wind Velocity : Inport  Port=2  Unit=m/s  PortDimensions=3
  Air Density : Inport  Port=3  Unit=kg/m^3
  Wind Angular Rates : Inport  Port=4  Unit=rad/s  PortDimensions=3
  Vb : Inport  Port=5  Unit=m/second  PortDimensions=3
  p,q,r : Inport  Port=6  Unit=rad/s  PortDimensions=3
  Dynamic Pressure : aerolibasang/Dynamic Pressure
  "Incidence, Sideslip & Airspeed" : aerolibasang/Incidence, Sideslip, & Airspeed
  Mach Number : aerolibasang/Mach Number
  Mux : Mux  Inputs=2
  Sum : Sum  Inputs=|+-  InputSameDT=on  SaturateOnIntegerOverflow=on  OutDataTypeStr=Inherit: Same as first input
  Sum1 : Sum  Inputs=|++  InputSameDT=on  SaturateOnIntegerOverflow=on  OutDataTypeStr=Inherit: Same as first input
  qbar : Outport  Unit=Pa  InitialOutput=0  VectorParamsAs1DForOutWhenUnconnected=off
  "p,q,r " : Outport  Port=2  Unit=rad/s  VectorParamsAs1DForOutWhenUnconnected=off
  V : Outport  Port=3  Unit=m/s  VectorParamsAs1DForOutWhenUnconnected=off
  Mach : Outport  Port=4  VectorParamsAs1DForOutWhenUnconnected=off
  Incid : Outport  Port=5  Unit=rad  VectorParamsAs1DForOutWhenUnconnected=off
  wires:
  Sum1/1 -> "p,q,r "/1
  Wind Angular Rates/1 -> Sum1/2
  p,q,r/1 -> Sum1/1
  "Incidence, Sideslip & Airspeed"/1 -> Mux/1  "Alpha"
  Mux/1 -> Incid/1
  "Incidence, Sideslip & Airspeed"/2 -> Mux/2  "Beta"
  Wind Velocity/1 -> Sum/2
  Speed of Sound/1 -> Mach Number/2
  Vb/1 -> Sum/1
  Sum/1 -> "Incidence, Sideslip & Airspeed"/1, Mach Number/1, Dynamic Pressure/1
  Mach Number/1 -> Mach/1
  Air Density/1 -> Dynamic Pressure/2
  Dynamic Pressure/1 -> qbar/1
  "Incidence, Sideslip & Airspeed"/3 -> V/1

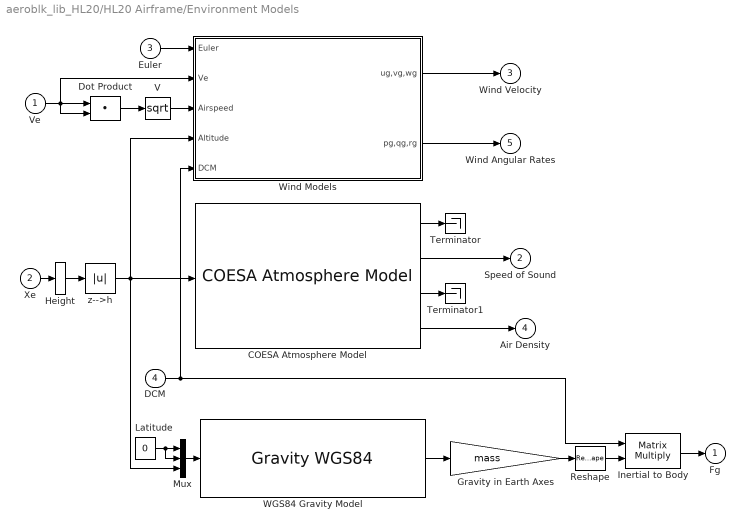
== system aeroblk_lib_HL20/HL20 Airframe/Environment Models ==
  Ve : Inport  Unit=m/s
  Xe : Inport  Port=2  Unit=meter  PortDimensions=3
  Euler : Inport  Port=3  Unit=rad
  DCM : Inport  Port=4
  COESA Atmosphere Model : aerolibatmos2/COESA Atmosphere Model  units=Metric (MKS)  spec=1976 COESA-extended U.S. Standard Atmosphere  model=Profile  profile_var=High temperature  profile_percent=10%  profile_alt=5 km (16404 ft)  envelope_var=High temperature  envelope_percent=1%  action=None
  Dot Product : DotProduct  SaturateOnIntegerOverflow=on  InputSameDT=off  OutDataTypeStr=Inherit: Inherit via internal rule
  Gravity in Earth Axes : Gain  Gain=mass  SaturateOnIntegerOverflow=on  OutDataTypeStr=Inherit: Same as input  ParamDataTypeStr=Inherit: Same as input
  Height : Selector  InputPortWidth=3  IndexOptions=Index vector (dialog)  Indices=[3]  OutputSizes=1
  Inertial to Body : Product  Multiplication=Matrix(*)  InputSameDT=on  SaturateOnIntegerOverflow=on  OutDataTypeStr=Inherit: Same as first input
  Latitude : Constant  Value=0
  Mux : Mux  Inputs=3
  Reshape : Reshape
  Terminator : Terminator
  Terminator1 : Terminator
  V : Math  Operator=sqrt  SignedPower=on
  "WGS84 Gravity Model  " : GravityWGS84  action=None
  Wind Models : Subsystem
  z-->h : Abs
  Fg : Outport  Unit=N  InitialOutput=0  VectorParamsAs1DForOutWhenUnconnected=off
  Speed of Sound : Outport  Port=2  Unit=m/second  InitialOutput=0  VectorParamsAs1DForOutWhenUnconnected=off
  Wind Velocity : Outport  Port=3  Unit=m/second  InitialOutput=0  VectorParamsAs1DForOutWhenUnconnected=off
  Air Density : Outport  Port=4  Unit=kg/m^3  InitialOutput=0  VectorParamsAs1DForOutWhenUnconnected=off
  Wind Angular Rates : Outport  Port=5  Unit=rad/second  InitialOutput=0  VectorParamsAs1DForOutWhenUnconnected=off
  wires:
  V/1 -> Wind Models/3(Airspeed)
  Inertial to Body/1 -> Fg/1
  DCM/1 -> Inertial to Body/1, Wind Models/5(DCM)
  Gravity in Earth Axes/1 -> Reshape/1
  "WGS84 Gravity Model  "/1 -> Gravity in Earth Axes/1
  Latitude/1 -> Mux/1, Mux/2
  Xe/1 -> Height/1
  Height/1 -> z-->h/1
  COESA Atmosphere Model/1 -> Terminator/1
  COESA Atmosphere Model/3 -> Terminator1/1
  COESA Atmosphere Model/2 -> Speed of Sound/1
  COESA Atmosphere Model/4 -> Air Density/1
  z-->h/1 -> Wind Models/4(Altitude), COESA Atmosphere Model/1, Mux/3
  Dot Product/1 -> V/1
  Wind Models/2(pg,qg,rg) -> Wind Angular Rates/1
  Wind Models/1(ug,vg,wg) -> Wind Velocity/1
  Ve/1 -> Dot Product/1, Wind Models/2(Ve), Dot Product/2
  Euler/1 -> Wind Models/1(Euler)
  Mux/1 -> "WGS84 Gravity Model  "/1
  Reshape/1 -> Inertial to Body/2

== system aeroblk_lib_HL20/HL20 Airframe/Forces and Moments ==
  Coeff : Inport
  Thrust : Inport  Port=2  Unit=N
  qbar : Inport  Port=3  Unit=Pa
  Aerodynamic Forces and Moments : aerolibadyn/Aerodynamic Forces and Moments   inputAxes=Body  outputForceAxes=Body  outputMomentAxes=Body  S=S_ref  b=b_ref  cbar=d_ref
  Center of Gravity : Constant  Value=[-x_cg 0 0]
  Center of Pressure : Constant  Value=[- x_ref 0 0]
  Sum : Sum  Inputs=++|  InputSameDT=on  SaturateOnIntegerOverflow=on  OutDataTypeStr=Inherit: Same as first input
  X,Y,Z : Outport  Unit=N  InitialOutput=0  VectorParamsAs1DForOutWhenUnconnected=off
  LMN : Outport  Port=2  Unit=N*m  InitialOutput=0  VectorParamsAs1DForOutWhenUnconnected=off
  wires:
  Coeff/1 -> Aerodynamic Forces and Moments/1
  qbar/1 -> Aerodynamic Forces and Moments/2
  Thrust/1 -> Sum/1
  Sum/1 -> X,Y,Z/1
  Aerodynamic Forces and Moments/2 -> LMN/1
  Aerodynamic Forces and Moments/1 -> Sum/2
  Center of Gravity/1 -> Aerodynamic Forces and Moments/3
  Center of Pressure/1 -> Aerodynamic Forces and Moments/4

== system aeroblk_lib_HL20/HL20 Airframe/Aerodynamic Coefficients/Actuator Increments ==
  Alpha : Inport  Unit=deg
  Beta : Inport  Port=2  Unit=deg
  "Actuator Deflections " : Inport  Port=3  Unit=deg
  (0 to inf) Constants Held fixed for alpha<0 : Saturate  UpperLimit=inf  LowerLimit=0
  Aileron : Subsystem
  AlphaLookup : PreLookup  BreakpointsData=alpha_vec_0  BeginIndexSearchUsingPreviousIndexResult=on  ExtrapMethod=Linear
  AlphaLookup0 : PreLookup  BreakpointsData=alpha_vec_0  BeginIndexSearchUsingPreviousIndexResult=on  ExtrapMethod=Linear
  Bus Creator : BusCreator  Inputs=2
  Bus Creator1 : BusCreator  Inputs=2
  Elevator : Subsystem
  Flap(diff) : Subsystem
  Flap(neg) : Subsystem
  Flap(pos) : Subsystem
  Rudder : Subsystem
  Sum : Sum  Inputs=++++++  InputSameDT=on  SaturateOnIntegerOverflow=on  OutDataTypeStr=Inherit: Same as first input
  Terminator1 : Terminator
  cl : Outport  InitialOutput=0  VectorParamsAs1DForOutWhenUnconnected=off
  wires:
  Bus Creator/1 -> Aileron/1(Alpha), Rudder/1(Alpha)
  (0 to inf) Constants Held fixed for alpha<0/1 -> AlphaLookup0/1
  "Actuator Deflections "/1 -> Aileron/2(Actuators), Elevator/2(Actuators), Rudder/2(Actuators), Flap(pos)/2(Actuators), Flap(neg)/2(Actuators), Flap(diff)/2(Actuators)
  Alpha/1 -> (0 to inf) Constants Held fixed for alpha<0/1, AlphaLookup/1
  Beta/1 -> Terminator1/1
  Aileron/1(delCoeff) -> Sum/1
  Elevator/1(delCoeff) -> Sum/2
  Rudder/1(delCoeff) -> Sum/3
  Flap(pos)/1(delCoeff) -> Sum/4
  Flap(neg)/1(delCoeff) -> Sum/5
  Flap(diff)/1(delCoeff) -> Sum/6
  Sum/1 -> cl/1
  Bus Creator1/1 -> Flap(diff)/1(Alpha), Flap(neg)/1(Alpha), Flap(pos)/1(Alpha), Elevator/1(Alpha)
  AlphaLookup0/1 -> Bus Creator/1  "k"
  AlphaLookup0/2 -> Bus Creator/2  "f"
  AlphaLookup/1 -> Bus Creator1/1  "k"
  AlphaLookup/2 -> Bus Creator1/2  "f"

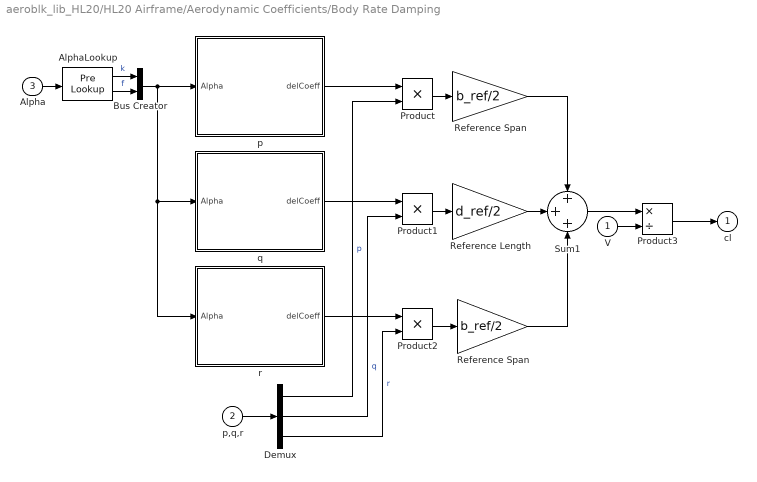
== system aeroblk_lib_HL20/HL20 Airframe/Aerodynamic Coefficients/Body Rate Damping ==
  V : Inport  Unit=m/s
  p,q,r : Inport  Port=2  Unit=rad/second
  Alpha : Inport  Port=3  Unit=deg
  AlphaLookup : PreLookup  BreakpointsData=alpha_vec_damping  BeginIndexSearchUsingPreviousIndexResult=on  ExtrapMethod=Linear
  Bus Creator : BusCreator  Inputs=2
  Demux : Demux  Outputs=3
      settings: DisplayOption=none
  Product : Product  InputSameDT=on  SaturateOnIntegerOverflow=on  OutDataTypeStr=Inherit: Same as first input
  Product1 : Product  InputSameDT=on  SaturateOnIntegerOverflow=on  OutDataTypeStr=Inherit: Same as first input
  Product2 : Product  InputSameDT=on  SaturateOnIntegerOverflow=on  OutDataTypeStr=Inherit: Same as first input
  Product3 : Product  Inputs=*/  InputSameDT=on  SaturateOnIntegerOverflow=on  OutDataTypeStr=Inherit: Same as first input
  Reference Length : Gain  Gain=d_ref/2  SaturateOnIntegerOverflow=on  OutDataTypeStr=Inherit: Same as input  ParamDataTypeStr=Inherit: Same as input
  Reference Span : Gain  Gain=b_ref/2  SaturateOnIntegerOverflow=on  OutDataTypeStr=Inherit: Same as input  ParamDataTypeStr=Inherit: Same as input
  "Reference Span " : Gain  Gain=b_ref/2  SaturateOnIntegerOverflow=on  OutDataTypeStr=Inherit: Same as input  ParamDataTypeStr=Inherit: Same as input
  Sum1 : Sum  Inputs=+++  InputSameDT=on  SaturateOnIntegerOverflow=on  OutDataTypeStr=Inherit: Same as first input
  p : Subsystem
  q : Subsystem
  r : Subsystem
  cl : Outport  InitialOutput=0  VectorParamsAs1DForOutWhenUnconnected=off
  wires:
  Alpha/1 -> AlphaLookup/1
  p/1(delCoeff) -> Product/1
  q/1(delCoeff) -> Product1/1
  p,q,r/1 -> Demux/1
  Demux/1 -> Product/2  "p"
  Demux/2 -> Product1/2  "q"
  Demux/3 -> Product2/2  "r"
  Sum1/1 -> Product3/1
  V/1 -> Product3/2
  Product3/1 -> cl/1
  Product1/1 -> Reference Length/1
  Product2/1 -> "Reference Span "/1
  Product/1 -> Reference Span/1
  r/1(delCoeff) -> Product2/1
  Bus Creator/1 -> r/1(Alpha), q/1(Alpha), p/1(Alpha)
  Reference Length/1 -> Sum1/2
  Reference Span/1 -> Sum1/1
  "Reference Span "/1 -> Sum1/3
  AlphaLookup/1 -> Bus Creator/1  "k"
  AlphaLookup/2 -> Bus Creator/2  "f"

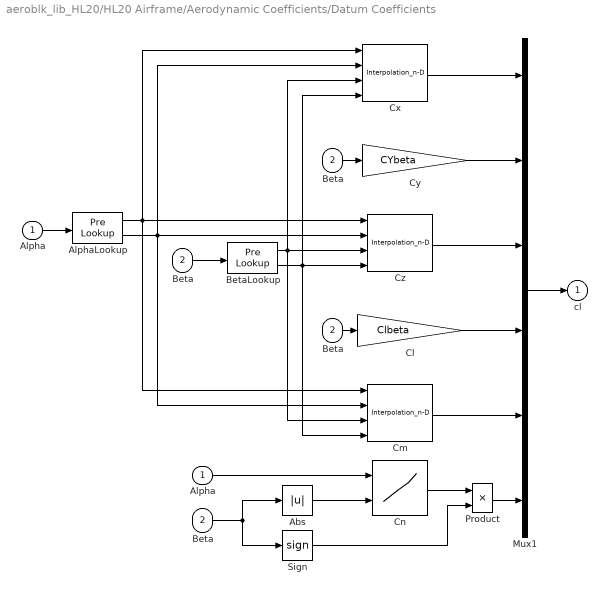
== system aeroblk_lib_HL20/HL20 Airframe/Aerodynamic Coefficients/Datum Coefficients ==
  Alpha : Inport  Unit=deg
  Beta : Inport  Port=2  Unit=deg
  " Cn" : Lookup_n-D  BreakpointsForDimension1=alpha_vec_Cn0  BreakpointsForDimension2=beta_vec_Cn0  Table=Cn0  InternalRulePriority=Speed  RndMeth=Simplest
      settings: InputPortMap=u0,u1
  " Beta" : InportShadow  Port=2  Unit=deg
  " Beta " : InportShadow  Port=2  Unit=deg
  Abs : Abs
  "Alpha " : InportShadow  Unit=deg
  AlphaLookup : PreLookup  BreakpointsData=alpha_vec_0  BeginIndexSearchUsingPreviousIndexResult=on  ExtrapMethod=Linear
  "Beta " : InportShadow  Port=2  Unit=deg
  BetaLookup : PreLookup  BreakpointsData=beta_vec_0  BeginIndexSearchUsingPreviousIndexResult=on  ExtrapMethod=Linear
  Cl : Gain  Gain=Clbeta  SaturateOnIntegerOverflow=on  OutDataTypeStr=Inherit: Same as input  ParamDataTypeStr=Inherit: Same as input
  Cm : Interpolation_n-D  Table=Cm0'  RemoveProtectionIndex=on
  Cx : Interpolation_n-D  Table=CX0'  RemoveProtectionIndex=on
  Cy : Gain  Gain=CYbeta  SaturateOnIntegerOverflow=on  OutDataTypeStr=Inherit: Same as input  ParamDataTypeStr=Inherit: Same as input
  Cz : Interpolation_n-D  Table=CZ0'  RemoveProtectionIndex=on
  Mux1 : Mux  Inputs=6
  Product : Product  InputSameDT=on  SaturateOnIntegerOverflow=on  OutDataTypeStr=Inherit: Same as first input
  Sign : Signum
  cl : Outport  InitialOutput=0  VectorParamsAs1DForOutWhenUnconnected=off
  wires:
  Sign/1 -> Product/2
  " Cn"/1 -> Product/1
  Product/1 -> Mux1/6
  Abs/1 -> " Cn"/2
  Mux1/1 -> cl/1
  Cx/1 -> Mux1/1
  Cz/1 -> Mux1/3
  Cm/1 -> Mux1/5
  Cy/1 -> Mux1/2
  Cl/1 -> Mux1/4
  Alpha/1 -> AlphaLookup/1
  Beta/1 -> BetaLookup/1
  AlphaLookup/1 -> Cz/1, Cm/1, Cx/1
  BetaLookup/1 -> Cz/3, Cx/3, Cm/3
  AlphaLookup/2 -> Cx/2, Cm/2, Cz/2
  "Beta "/1 -> Cy/1
  "Alpha "/1 -> " Cn"/1
  " Beta"/1 -> Abs/1, Sign/1
  " Beta "/1 -> Cl/1
  BetaLookup/2 -> Cz/4, Cx/4, Cm/4

== system aeroblk_lib_HL20/HL20 Airframe/Environment Models/Wind Models ==
  Euler : Inport  Unit=rad
  Ve : Inport  Port=2  Unit=m/s
  Airspeed : Inport  Port=3  Unit=m/s
  Altitude : Inport  Port=4  Unit=m
  DCM : Inport  Port=5
  Discrete Wind Gust Model - On : aerolibwind2/Discrete Wind Gust Model  units=Metric (MKS)  Gx=on  Gy=on  Gz=on  t_0=20  d_m=[120 120 80]  v_m=[3.5 3.0 3.0]
  Dryden Wind Turbulence Model (Continuous (+q -r)) : aerolibwind2/Dryden Wind Turbulence Model  (Continuous (+q -r))  units=Metric (MKS)  spec=MIL-F-8785C  model=Continuous Dryden (+q -r)  W20=5  Wdeg=0  TurbProb=10^-2 - Light  L_high=533.4  Wingspan=4  ts=0.1  Seed=[23341 23342 23343 23344]  T_on=on
  Sum : Sum  Inputs=+++  InputSameDT=on  SaturateOnIntegerOverflow=on  OutDataTypeStr=Inherit: Same as first input
  Terminator : Terminator
  Terminator1 : Terminator
  Wind Shear Model : aerolibwind2/Wind Shear Model  units=Metric (MKS)  phase=Category C - Terminal Flight Phase  W_20=1  Wdeg=0
  ug,vg,wg : Outport  Unit=m/s  VectorParamsAs1DForOutWhenUnconnected=off
  pg,qg,rg : Outport  Port=2  Unit=rad/s  VectorParamsAs1DForOutWhenUnconnected=off
  wires:
  Altitude/1 -> Wind Shear Model/1, Dryden Wind Turbulence Model (Continuous (+q -r))/1
  Dryden Wind Turbulence Model (Continuous (+q -r))/2 -> pg,qg,rg/1
  Airspeed/1 -> Discrete Wind Gust Model - On/1, Dryden Wind Turbulence Model (Continuous (+q -r))/2
  DCM/1 -> Wind Shear Model/2, Dryden Wind Turbulence Model (Continuous (+q -r))/3
  Sum/1 -> ug,vg,wg/1
  Discrete Wind Gust Model - On/1 -> Sum/3
  Dryden Wind Turbulence Model (Continuous (+q -r))/1 -> Sum/2
  Wind Shear Model/1 -> Sum/1
  Ve/1 -> Terminator/1
  Euler/1 -> Terminator1/1

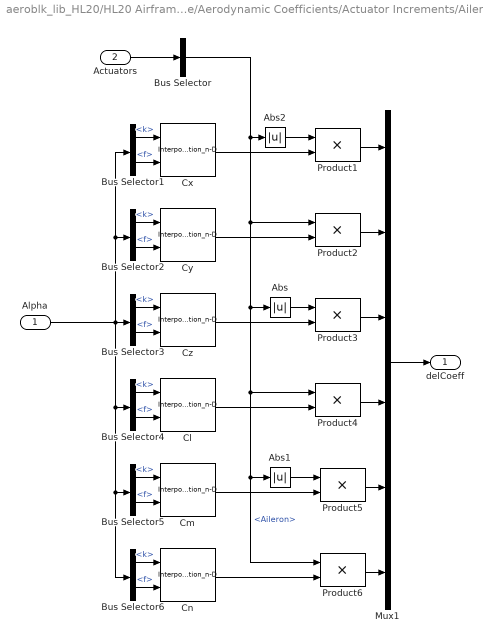
== system aeroblk_lib_HL20/HL20 Airframe/Aerodynamic Coefficients/Actuator Increments/Aileron ==
  Alpha : Inport
  Actuators : Inport  Port=2
  Abs : Abs
  Abs1 : Abs
  Abs2 : Abs
  Bus Selector : BusSelector  OutputSignals=Aileron
  Bus Selector{1..6} (6 alike) : BusSelector  OutputSignals=k,f
  Cl : Interpolation_n-D  NumberOfTableDimensions=1  Table=Clda  RemoveProtectionIndex=on
      settings: InputPortMap=u0,u1
  Cm : Interpolation_n-D  NumberOfTableDimensions=1  Table=Cmda  RemoveProtectionIndex=on
      settings: InputPortMap=u0,u1
  Cn : Interpolation_n-D  NumberOfTableDimensions=1  Table=Cnda  RemoveProtectionIndex=on
      settings: InputPortMap=u0,u1
  Cx : Interpolation_n-D  NumberOfTableDimensions=1  Table=CXda  RemoveProtectionIndex=on
      settings: InputPortMap=u0,u1
  Cy : Interpolation_n-D  NumberOfTableDimensions=1  Table=CYda  RemoveProtectionIndex=on
      settings: InputPortMap=u0,u1
  Cz : Interpolation_n-D  NumberOfTableDimensions=1  Table=CZda  RemoveProtectionIndex=on
      settings: InputPortMap=u0,u1
  Mux1 : Mux  Inputs=6
  Product{1..6} (6 alike) : Product  InputSameDT=on  SaturateOnIntegerOverflow=on  OutDataTypeStr=Inherit: Same as first input
  delCoeff : Outport  VectorParamsAs1DForOutWhenUnconnected=off
  wires:
  Actuators/1 -> Bus Selector/1
  Mux1/1 -> delCoeff/1
  Product1/1 -> Mux1/1
  Cx/1 -> Product1/2
  Product2/1 -> Mux1/2
  Cy/1 -> Product2/2
  Product3/1 -> Mux1/3
  Cz/1 -> Product3/2
  Cl/1 -> Product4/2
  Product4/1 -> Mux1/4
  Cm/1 -> Product5/2
  Product5/1 -> Mux1/5
  Cn/1 -> Product6/2
  Product6/1 -> Mux1/6
  Bus Selector/1 -> Product6/1, Abs1/1, Product4/1, Abs/1, Product2/1, Abs2/1  "<Aileron>"
  Abs/1 -> Product3/1
  Abs1/1 -> Product5/1
  Abs2/1 -> Product1/1
  Alpha/1 -> Bus Selector1/1, Bus Selector2/1, Bus Selector5/1, Bus Selector6/1, Bus Selector4/1, Bus Selector3/1
  Bus Selector1/1 -> Cx/1  "<k>"
  Bus Selector1/2 -> Cx/2  "<f>"
  Bus Selector2/1 -> Cy/1  "<k>"
  Bus Selector2/2 -> Cy/2  "<f>"
  Bus Selector3/1 -> Cz/1  "<k>"
  Bus Selector3/2 -> Cz/2  "<f>"
  Bus Selector4/1 -> Cl/1  "<k>"
  Bus Selector4/2 -> Cl/2  "<f>"
  Bus Selector5/1 -> Cm/1  "<k>"
  Bus Selector5/2 -> Cm/2  "<f>"
  Bus Selector6/1 -> Cn/1  "<k>"
  Bus Selector6/2 -> Cn/2  "<f>"

== system aeroblk_lib_HL20/HL20 Airframe/Aerodynamic Coefficients/Actuator Increments/Elevator ==
  Alpha : Inport
  Actuators : Inport  Port=2
  Bus Selector1 : BusSelector  OutputSignals=Elevator
  Bus Selector2 : BusSelector  OutputSignals=k,f
  Bus Selector3 : BusSelector  OutputSignals=k,f
  Bus Selector5 : BusSelector  OutputSignals=k,f
  Cm : Interpolation_n-D  NumberOfTableDimensions=1  Table=Cmde  RemoveProtectionIndex=on
      settings: InputPortMap=u0,u1
  Constant1 : Constant  Value=0
  Cx : Interpolation_n-D  NumberOfTableDimensions=1  Table=CXde  RemoveProtectionIndex=on
      settings: InputPortMap=u0,u1
  Cz : Interpolation_n-D  NumberOfTableDimensions=1  Table=CZde  RemoveProtectionIndex=on
      settings: InputPortMap=u0,u1
  Mux1 : Mux  Inputs=6
  Product : Product  InputSameDT=on  SaturateOnIntegerOverflow=on  OutDataTypeStr=Inherit: Same as first input
  delCoeff : Outport  VectorParamsAs1DForOutWhenUnconnected=off
  wires:
  Product/1 -> delCoeff/1
  Mux1/1 -> Product/1
  Alpha/1 -> Bus Selector2/1, Bus Selector3/1, Bus Selector5/1
  Cx/1 -> Mux1/1
  Cz/1 -> Mux1/3
  Cm/1 -> Mux1/5
  Constant1/1 -> Mux1/2, Mux1/4, Mux1/6
  Actuators/1 -> Bus Selector1/1
  Bus Selector1/1 -> Product/2  "<Elevator>"
  Bus Selector2/1 -> Cx/1  "<k>"
  Bus Selector2/2 -> Cx/2  "<f>"
  Bus Selector3/1 -> Cz/1  "<k>"
  Bus Selector3/2 -> Cz/2  "<f>"
  Bus Selector5/1 -> Cm/1  "<k>"
  Bus Selector5/2 -> Cm/2  "<f>"

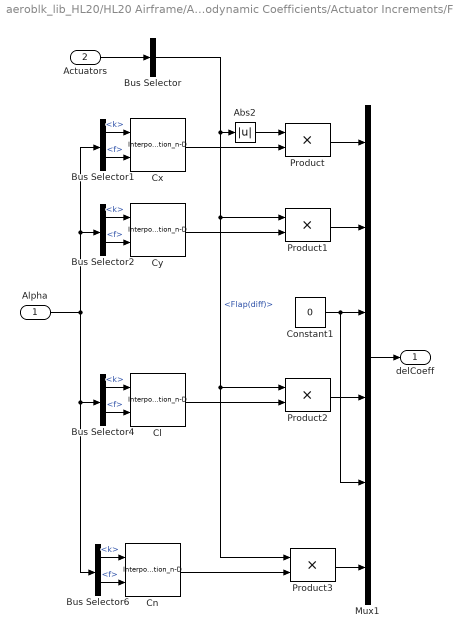
== system aeroblk_lib_HL20/HL20 Airframe/Aerodynamic Coefficients/Actuator Increments/Flap(diff) ==
  Alpha : Inport
  Actuators : Inport  Port=2
  Abs2 : Abs
  Bus Selector : BusSelector  OutputSignals=Flap(diff)
  Bus Selector{1..2,4,6} (4 alike) : BusSelector  OutputSignals=k,f
  Cl : Interpolation_n-D  NumberOfTableDimensions=1  Table=Clddf  RemoveProtectionIndex=on
      settings: InputPortMap=u0,u1
  Cn : Interpolation_n-D  NumberOfTableDimensions=1  Table=Cnddf  RemoveProtectionIndex=on
      settings: InputPortMap=u0,u1
  Constant1 : Constant  Value=0
  Cx : Interpolation_n-D  NumberOfTableDimensions=1  Table=CXddf  RemoveProtectionIndex=on
      settings: InputPortMap=u0,u1
  Cy : Interpolation_n-D  NumberOfTableDimensions=1  Table=CYddf  RemoveProtectionIndex=on
      settings: InputPortMap=u0,u1
  Mux1 : Mux  Inputs=6
  Product{,1..3} (4 alike) : Product  InputSameDT=on  SaturateOnIntegerOverflow=on  OutDataTypeStr=Inherit: Same as first input
  delCoeff : Outport  VectorParamsAs1DForOutWhenUnconnected=off
  wires:
  Mux1/1 -> delCoeff/1
  Alpha/1 -> Bus Selector4/1, Bus Selector6/1, Bus Selector1/1, Bus Selector2/1
  Actuators/1 -> Bus Selector/1
  Product/1 -> Mux1/1
  Cx/1 -> Product/2
  Bus Selector/1 -> Product3/1, Product2/1, Product1/1, Abs2/1  "<Flap(diff)>"
  Product1/1 -> Mux1/2
  Product2/1 -> Mux1/4
  Cl/1 -> Product2/2
  Cy/1 -> Product1/2
  Product3/1 -> Mux1/6
  Cn/1 -> Product3/2
  Abs2/1 -> Product/1
  Constant1/1 -> Mux1/3, Mux1/5
  Bus Selector1/1 -> Cx/1  "<k>"
  Bus Selector1/2 -> Cx/2  "<f>"
  Bus Selector2/1 -> Cy/1  "<k>"
  Bus Selector2/2 -> Cy/2  "<f>"
  Bus Selector4/1 -> Cl/1  "<k>"
  Bus Selector4/2 -> Cl/2  "<f>"
  Bus Selector6/1 -> Cn/1  "<k>"
  Bus Selector6/2 -> Cn/2  "<f>"

== system aeroblk_lib_HL20/HL20 Airframe/Aerodynamic Coefficients/Actuator Increments/Flap(neg) ==
  Alpha : Inport
  Actuators : Inport  Port=2
  Bus Selector : BusSelector  OutputSignals=Flap(neg)
  Bus Selector1 : BusSelector  OutputSignals=k,f
  Bus Selector3 : BusSelector  OutputSignals=k,f
  Bus Selector5 : BusSelector  OutputSignals=k,f
  Cm : Interpolation_n-D  NumberOfTableDimensions=1  Table=Cmdfn  RemoveProtectionIndex=on
      settings: InputPortMap=u0,u1
  Constant1 : Constant  Value=0
  Constant2 : Constant  Value=0
  Constant3 : Constant  Value=0
  Cx : Interpolation_n-D  NumberOfTableDimensions=1  Table=CXdfn  RemoveProtectionIndex=on
      settings: InputPortMap=u0,u1
  Cz : Interpolation_n-D  NumberOfTableDimensions=1  Table=CZdfn  RemoveProtectionIndex=on
      settings: InputPortMap=u0,u1
  Mux1 : Mux  Inputs=6
  Product : Product  InputSameDT=on  SaturateOnIntegerOverflow=on  OutDataTypeStr=Inherit: Same as first input
  delCoeff : Outport  VectorParamsAs1DForOutWhenUnconnected=off
  wires:
  Cm/1 -> Mux1/5
  Cz/1 -> Mux1/3
  Cx/1 -> Mux1/1
  Alpha/1 -> Bus Selector5/1, Bus Selector3/1, Bus Selector1/1
  Mux1/1 -> Product/1
  Product/1 -> delCoeff/1
  Actuators/1 -> Bus Selector/1
  Constant1/1 -> Mux1/2
  Constant2/1 -> Mux1/4
  Constant3/1 -> Mux1/6
  Bus Selector/1 -> Product/2  "<Flap(neg)>"
  Bus Selector5/1 -> Cm/1  "<k>"
  Bus Selector5/2 -> Cm/2  "<f>"
  Bus Selector3/1 -> Cz/1  "<k>"
  Bus Selector3/2 -> Cz/2  "<f>"
  Bus Selector1/1 -> Cx/1  "<k>"
  Bus Selector1/2 -> Cx/2  "<f>"

== system aeroblk_lib_HL20/HL20 Airframe/Aerodynamic Coefficients/Actuator Increments/Flap(pos) ==
  Alpha : Inport
  Actuators : Inport  Port=2
  Bus Selector : BusSelector  OutputSignals=Flap(pos)
  Bus Selector1 : BusSelector  OutputSignals=k,f
  Bus Selector3 : BusSelector  OutputSignals=k,f
  Bus Selector5 : BusSelector  OutputSignals=k,f
  Cm : Interpolation_n-D  NumberOfTableDimensions=1  Table=Cmdfp  RemoveProtectionIndex=on
      settings: InputPortMap=u0,u1
  Constant1 : Constant  Value=0
  Constant2 : Constant  Value=0
  Constant3 : Constant  Value=0
  Cx : Interpolation_n-D  NumberOfTableDimensions=1  Table=CXdfp  RemoveProtectionIndex=on
      settings: InputPortMap=u0,u1
  Cz : Interpolation_n-D  NumberOfTableDimensions=1  Table=CZdfp  RemoveProtectionIndex=on
      settings: InputPortMap=u0,u1
  Mux1 : Mux  Inputs=6
  Product : Product  InputSameDT=on  SaturateOnIntegerOverflow=on  OutDataTypeStr=Inherit: Same as first input
  delCoeff : Outport  VectorParamsAs1DForOutWhenUnconnected=off
  wires:
  Product/1 -> delCoeff/1
  Mux1/1 -> Product/1
  Alpha/1 -> Bus Selector5/1, Bus Selector3/1, Bus Selector1/1
  Cx/1 -> Mux1/1
  Cz/1 -> Mux1/3
  Cm/1 -> Mux1/5
  Constant1/1 -> Mux1/2
  Constant2/1 -> Mux1/4
  Constant3/1 -> Mux1/6
  Actuators/1 -> Bus Selector/1
  Bus Selector/1 -> Product/2  "<Flap(pos)>"
  Bus Selector5/1 -> Cm/1  "<k>"
  Bus Selector5/2 -> Cm/2  "<f>"
  Bus Selector3/1 -> Cz/1  "<k>"
  Bus Selector3/2 -> Cz/2  "<f>"
  Bus Selector1/1 -> Cx/1  "<k>"
  Bus Selector1/2 -> Cx/2  "<f>"
